simulink model "TO_Roll"  (R2025b)
settings: Solver=VariableStepAuto  StartTime=0.0  StopTime=tFinal  RelTol=1e-3
values from neighbouring files (symbols this model uses):
  CD = 0.04    [initTO.m]
  CL = 1.8    [initTO.m]
  m = 6000    [initTO.m]
  mu_roll = 0.02    [initTO.m]
  rho = 1.225    [initTO.m]
  S = 30    [initTO.m]
  T = T_over_W * W    (= 20601)    [initTO.m]
  V_to = 1.2 * Vs    [initTO.m]
  W = m * g    (= 58860)    [initTO.m]
libraries: simulink x1

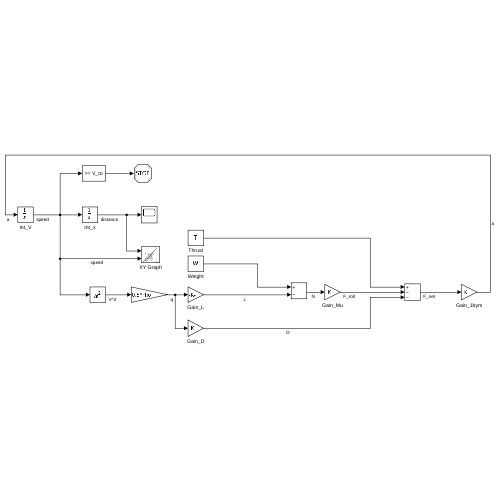
[thumbnail: Simulink's stored preview of the top-level diagram]
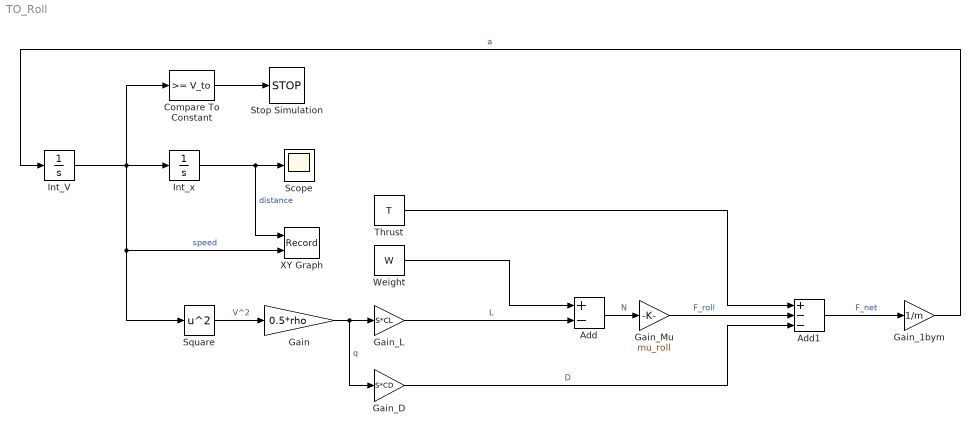
== system TO_Roll ==
  Add : Sum  Inputs=+-
  Add1 : Sum  Inputs=+--
  Compare To Constant : simulink/Logic and Bit Operations/Compare To Constant  relop=>=  const=V_to  OutDataTypeStr=boolean
  Gain : Gain  Gain=0.5*rho
  Gain_1bym : Gain  Gain=1/m
  Gain_D : Gain  Gain=S*CD
  Gain_L : Gain  Gain=S*CL
  Gain_Mu : Gain  Gain=mu_roll
  Int_V : Integrator
  Int_x : Integrator
  Scope : Scope
      settings: ActiveDisplayYMinimum=-49.715772829989604  ActiveDisplayYMaximum=447.44195546990659
  Square : Math  Operator=square
  Stop Simulation : Stop
  Thrust : Constant  Value=T
  Weight : Constant  Value=W
  XY Graph : Record  NumPorts=2.0  FileSettingsInternal="{\"entries\":[{\"content\":{\"excelSettings\":{\"content\":{},\"type\":\"Streamout.ExcelSettings\"},\"parquetSettings\":{\"content\":{},\"type\":\"Streamout.ParquetSettings\"}},\"type\":\"Streamout.FileSettingStorage\",\"uuid\":\"\"}],\"packageUris\":[\"http:\\/\\/schema.mathworks.com\\/mf0\\/streamout_blocks\\/R2020a\"],\"version\":\"1.0\"}"  FrameSettings=[0, 0]  Layout=[1 1]  SignalsInternal="{\"entries\":[{\"content\":{\"signals\":[{\"content\":{\"blockPath\":[],\"dimensions\":[1],\"domain\":\"\",\"lineColor\":\"#a2142f\",\"plots\":[ 1 ],\"port\":1,\"sid\":[\"\"],\"signalID\":1,\"signalName\":\"distance\"},\"type\":\"RecordBlkView.Signal\",\"uuid\":\"\"},{\"content\":{\"blockPath\":[],\"dimensions\":[1],\"domain\":\"\",\"lineColor\":\"#139fff\",\"plots\":[ 1 ],\"port\":2,\"sid\":[\"\"],\"signalID\":2,\"signalName\":\"speed\"},\"type\":\"RecordBlkView.Signal\",\"uuid\":\"\"}]},\"type\":\"RecordBlkView.InputSignals\",\"uuid\":\"\"}],\"packageUris\":[\"http:\\/\\/schema.mathworks.com\\/mf0\\/streamout_blocks\\/R2020a\"],\"version\":\"1.0\"}"  VisualizationBindings="{\"xyplotplugin\":{\"info\":[{\"series\":[{\"bindingParametersList\":[{\"parameter\":\"X-Axis\",\"signalID\":1,\"signalName\":\"distance\"},{\"parameter\":\"Y-Axis\",\"signalID\":2,\"signalName\":\"speed\"}],\"seriesID\":0}],\"subplotID\":1}]}}"  CompatibilityTag=XY
  wires:
  Int_V/1 -> XY Graph/2, Square/1, Int_x/1, Compare To Constant/1  "speed"
  Int_x/1 -> XY Graph/1, Scope/1  "distance"
  Square/1 -> Gain/1  "V^2"
  Gain/1 -> Gain_D/1, Gain_L/1  "q"
  Gain_L/1 -> Add/2  "L"
  Gain_D/1 -> Add1/3  "D"
  Weight/1 -> Add/1
  Add/1 -> Gain_Mu/1  "N"
  Gain_Mu/1 -> Add1/2  "F_roll"
  Thrust/1 -> Add1/1
  Add1/1 -> Gain_1bym/1  "F_net"
  Gain_1bym/1 -> Int_V/1  "a"
  Compare To Constant/1 -> Stop Simulation/1
